simulink model "MPPT_PO"  (R2018a)
settings: Solver=FixedStepDiscrete  StartTime=0.0  StopTime=800  FixedStep=5e-6  RelTol=1e-3
libraries: powerlib x10, re_lib x1
settings Model: Creator=yusuf  LastModifiedBy=yusuf

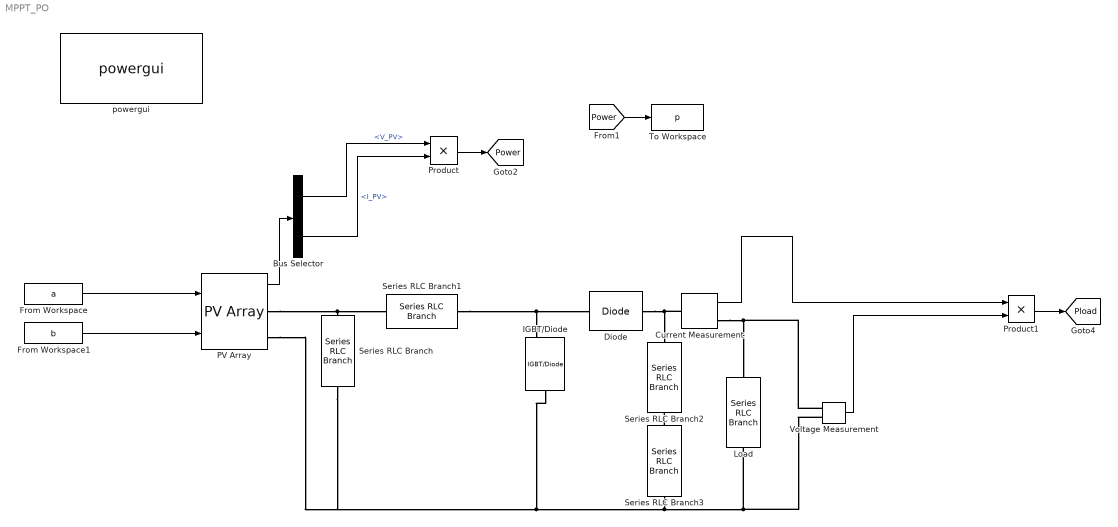
== system MPPT_PO ==
  Bus Selector : BusSelector  OutputSignals=V_PV,I_PV
  Current Measurement : powerlib/Measurements/Current Measurement  PhasorSimulation=off  OutputType=Complex  PSBequivalent=0
  Diode : powerlib/Power Electronics/Diode  Ron=0.001  Lon=0  Vf=0.8  IC=0  UseSnubber=0  Rs=500  Cs=250e-9  Measurements=off
  From Workspace : FromWorkspace  VariableName=a  SampleTime=1000000*(3e-6)
  From Workspace1 : FromWorkspace  VariableName=b  SampleTime=1000000*(3e-6)
  IGBT/Diode : powerlib/Power Electronics/IGBT//Diode  Ron=1e-3  Rs=1e5  Cs=inf  Measurements=off
  "Load " : powerlib/Elements/Series RLC Branch  LConnTagsString=__new0  RConnTagsString=__new0  BranchType=R  Resistance=10  Inductance=5e-3  SetiL0=off  InitialCurrent=0  Capacitance=12000e-6  Setx0=off  InitialVoltage=0  Measurements=None
  PV Array : re_lib/Solar/PV Array  Npar=64  Nser=5  PlotType=array @ 1000 W/m2 & specified temperatures  S_vec="[ 1000  500  100 ]"  Temp_C_vec="[ 35 45 55 65 75  ]"  ModuleName=MX Solar USA MX60-220  PlotWhenSelected=off  Pm=219.929  Ncell=60  Voc=36.5  Isc=8.24  Vm=28.9  Im=7.61  beta_Voc_pc=-0.36901  alpha_Isc_pc=0.087998  beta_Voc=-0.13469  alpha_Isc=0.007251  IL=8.2621  I0=3.9406e-10  nI=0.9975  Rsh=154.3792  Rs=0.41403  BAL=off  Tc=1e-6  Tfilter=5e-5
  Product : Product
  Product1 : Product
  Series RLC Branch : powerlib/Elements/Series RLC Branch  LConnTagsString=__new0  RConnTagsString=__new0  BranchType=C  Resistance=1  Inductance=1e-3  SetiL0=off  InitialCurrent=0  Capacitance=100e-3  Setx0=off  InitialVoltage=0  Measurements=None
  Series RLC Branch1 : powerlib/Elements/Series RLC Branch  LConnTagsString=__new0  RConnTagsString=__new0  BranchType=L  Resistance=1  Inductance=5e-3  SetiL0=off  InitialCurrent=0  Capacitance=100e-6  Setx0=off  InitialVoltage=0  Measurements=None
  Series RLC Branch2 : powerlib/Elements/Series RLC Branch  LConnTagsString=__new0  RConnTagsString=__new0  BranchType=C  Resistance=1  Inductance=5e-3  SetiL0=off  InitialCurrent=0  Capacitance=12000e-6  Setx0=off  InitialVoltage=0  Measurements=None
  Series RLC Branch3 : powerlib/Elements/Series RLC Branch  LConnTagsString=__new0  RConnTagsString=__new0  BranchType=C  Resistance=1  Inductance=5e-3  SetiL0=off  InitialCurrent=0  Capacitance=12000e-6  Setx0=off  InitialVoltage=0  Measurements=None
  To Workspace : ToWorkspace  VariableName=p  SaveFormat=Timeseries  SampleTime=0.1
  Voltage Measurement : powerlib/Measurements/Voltage Measurement  PhasorSimulation=off  OutputType=Complex  PSBequivalent=0
  powergui : powerlib/powergui  Priority=1  SimulationMode=Discrete  SampleTime=5e-6  frequency=60  Iterations=50  frequencyindice=0  Pbase=100e6  ErrMax=1e-4  UnitsV=kV  UnitsW=MW  buscounter=0  FunctionMessages=off  echomessages=off  EnableUseOfTLC=off  CurrentSourceSwitches=off  DisableSnubberDevices=off  DisableRonSwitches=off  DisableVfSwitches=off  DisplayEquations=off  SolverType=Tustin/Backward Euler (TBE)  Interpol=off  ExternalGateDelay=off  methode=off  Ts=100  x0status=blocks  SPID=off  SwTol=0  HookPort=off  RestoreLinks=warning  ResistiveCurrentMeasurement=off  Frange=[0:2:500]  Ylog=off  Xlog=on  ShowGrid=off  save=off  variable=ZData  structure=0  ZoomFFT=off  StartTime=0.0  cycles=1  DisplayStyle=1  fundamental=60  FreqAxis=off  MaxFrequency=1000  frequencyindicesteady=1  RmsSteady=1  display=off
  tag scope: Pload=global, Power=global
  wires:
  PV Array/1 -> Bus Selector/1
  Bus Selector/2 -> Product/2  "<I_PV>"
  Bus Selector/1 -> Product/1  "<V_PV>"
  Voltage Measurement/1 -> Product1/2
  From Workspace/1 -> PV Array/1
  From Workspace1/1 -> PV Array/2
  Product/1 -> [Power]
  [Power] -> To Workspace/1
  Product1/1 -> [Pload]
  Current Measurement/1 -> Product1/1
  connections:
  PV Array/RConn1 -- Series RLC Branch1/RConn1 -- Series RLC Branch/LConn1
  Series RLC Branch1/LConn1 -- Diode/LConn1 -- IGBT/Diode/LConn1
  Series RLC Branch3/RConn1 -- Series RLC Branch2/LConn1
  Voltage Measurement/LConn1 -- "Load "/RConn1 -- Current Measurement/RConn1
  Series RLC Branch3/LConn1 -- PV Array/RConn2 -- Series RLC Branch/RConn1 -- IGBT/Diode/RConn1 -- Voltage Measurement/LConn2 -- "Load "/LConn1
  Current Measurement/LConn1 -- Diode/RConn1 -- Series RLC Branch2/RConn1
